simulink model "untitled"  (Simulink 6.0)
settings: Solver=ode45  StartTime=0.0  StopTime=10.0  RelTol=1e-3
settings Model: LastModifiedBy=ntuser

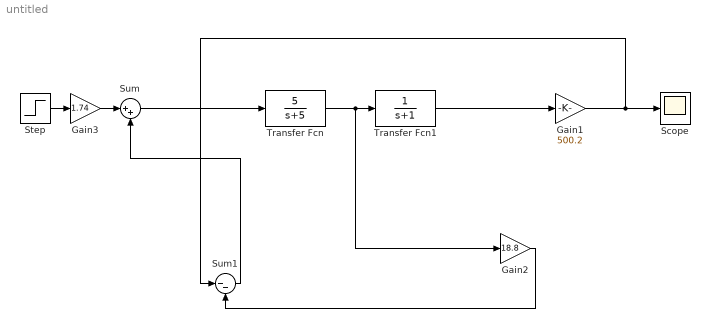
== system untitled ==
  Gain1 : Gain  Gain=500.2
  Gain2 : Gain  Gain=18.8
  Gain3 : Gain  Gain=1.74
  Scope : Scope
  Step : Step  After=3  SampleTime=0
  Sum : Sum  Inputs=|++
  Sum1 : Sum  Inputs=|--
  Transfer Fcn : TransferFcn  Numerator=[5]  Denominator=[1 5]
  Transfer Fcn1 : TransferFcn  Denominator=[1 1]
  wires:
  Step/1 -> Gain3/1
  Transfer Fcn/1 -> Transfer Fcn1/1, Gain2/1
  Transfer Fcn1/1 -> Gain1/1
  Gain1/1 -> Scope/1, Sum1/1
  Sum1/1 -> Sum/2
  Gain2/1 -> Sum1/2
  Sum/1 -> Transfer Fcn/1
  Gain3/1 -> Sum/1
